simulink model "sample_and_hold"  (R2015b)
settings: Solver=VariableStepAuto  StartTime=0.0  StopTime=10.0  RelTol=1e-3
values from neighbouring files (symbols this model uses):
  h = 2/10    (= 0.2)    [aliasing_example_model.m]    (also in notch_filter_example.m = 0.5; notch_filter_tustin_example.m = 0.5; sixty_hertz_hum_alias.m = 0.1)
settings Model: Creator=kjartan  LastModifiedBy=kjartan

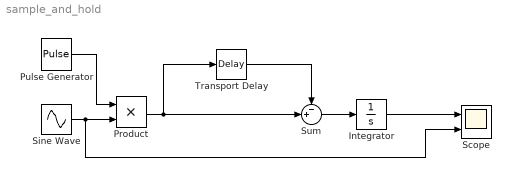
== system sample_and_hold ==
  Integrator : Integrator
  Product : Product
  Pulse Generator : DiscretePulseGenerator  PulseType=Time based  Amplitude=1/0.01  Period=h
  Scope : Scope  NumInputPorts=2
  Sine Wave : Sin  SampleTime=0
  Sum : Sum  Inputs=-+|
  Transport Delay : TransportDelay  DelayTime=h
  wires:
  Transport Delay/1 -> Sum/1
  Integrator/1 -> Scope/1
  Sum/1 -> Integrator/1
  Product/1 -> Transport Delay/1, Sum/2
  Sine Wave/1 -> Scope/2, Product/2
  Pulse Generator/1 -> Product/1
